simulink model "SNAP_DETUMBLE_HighPassFilter"  (R2024a)
settings: Solver=ode45  StartTime=0.0  StopTime=SNAP_sim_length  FixedStep=0.1  MaxStep=0.01  RelTol=1e-2  EnableMultiTasking=on
InitFcn:
  | SNAP_Simulink_Init_Function
values from neighbouring files (symbols this model uses):
  bias = [28.8675 28.8675 28.8675]    [SNAP_Simulink_Init_Function.m]    (also in Script_magnetorquer_and_magnetometer.m; SnapParameters.m)
  boira_Imax = boira_max_magnetic_torque./boira_magnetic_gains    [SNAP_Simulink_Init_Function.m]    (also in Script_magnetorquer_and_magnetometer.m; SnapParameters.m)
  boira_magnetic_gains = [2.3 2.3 2.1]    [SNAP_Simulink_Init_Function.m]    (also in Script_magnetorquer_and_magnetometer.m; SnapParameters.m)
  day = C - E + F - floor(30.6001 * G)    [julian2datetime.m]
  EN_2BodyModel = 1    [SNAP_Simulink_Init_Function.m]
  EN_Aero = SNAP_sim_params.aero_enabled    [SNAP_Simulink_Init_Function.m]
  EN_GG = 1    [SNAP_Simulink_Init_Function.m]
  EN_Hyst = 0    [SNAP_Simulink_Init_Function.m]
  EN_Mag = 1    [SNAP_Simulink_Init_Function.m]
  initial_position = SNAP_sim_params.initial_position    [SNAP_Simulink_Init_Function.m]
  initial_velocity = SNAP_sim_params.initial_velocity    [SNAP_Simulink_Init_Function.m]
  lookup_breakpoints_mmeter = linspace(-200,200,50)*10^3    [SNAP_Simulink_Init_Function.m]    (also in Script_magnetorquer_and_magnetometer.m; SnapParameters.m)
  lookup_breakpoints_mtorquer = linspace(-boira_Imax(1)*2,boira_Imax(1)*2,55)    [SNAP_Simulink_Init_Function.m]    (also in Script_magnetorquer_and_magnetometer.m; SnapParameters.m)
  lookup_tabledata_mmeter = lookup_breakpoints_mmeter+max_deviation_mmeter*sin(pi*lookup_breakpoints_mmeter/max_breakpoint_mmeter)    [SNAP_Simulink_Init_Function.m]    (also in Script_magnetorquer_and_magnetometer.m; SnapParameters.m)
  lookup_tabledata_mtorquer = lookup_breakpoints_mtorquer+max_deviation_mtorquer*sin(pi*lookup_breakpoints_mtorquer/max_breakpoint_mtorquer)    [SNAP_Simulink_Init_Function.m]    (also in Script_magnetorquer_and_magnetometer.m; SnapParameters.m)
  noise = 0    [SNAP_Simulink_Init_Function.m]    (also in Script_magnetorquer_and_magnetometer.m; SnapParameters.m)
  noise_variance = 30    [SNAP_Simulink_Init_Function.m]    (also in Script_magnetorquer_and_magnetometer.m; SnapParameters.m)
  rotm_mmeter = eul2rotm([missalingment_x_mmeter missalingment_y_mmeter missalingment_z_mmeter])    [SNAP_Simulink_Init_Function.m]    (also in Script_magnetorquer_and_magnetometer.m; SnapParameters.m)
  rotm_mtorquer = eul2rotm([missalingment_x_mtorquer missalingment_y_mtorquer missalingment_z_mtorquer])    [SNAP_Simulink_Init_Function.m]    (also in Script_magnetorquer_and_magnetometer.m; SnapParameters.m)
  second = (day_fraction - hour - minute / 60) * 3600    [julian2datetime.m]
  SNAP_Br = SNAP_sim_params.Br    [SNAP_Simulink_Init_Function.m]
  SNAP_Bs = SNAP_sim_params.Bs    [SNAP_Simulink_Init_Function.m]
  SNAP_CONST_a3H0 = 7.943e15    (= 7.943e+15)    [SNAP_Simulink_Init_Function.m]
  SNAP_CONST_earth_mag_dipole = [sin(168.6*pi/180)* cos(109.3*pi/180), sin(168.6*pi/180)* sin(109.3*pi/180), cos(168.6*pi/180)]    [SNAP_Simulink_Init_Function.m]
  SNAP_CONST_G_earth = 6.6742e-11    [SNAP_Simulink_Init_Function.m]
  SNAP_CONST_m_earth = 5.9736e24    (= 5.9736e+24)    [SNAP_Simulink_Init_Function.m]
  SNAP_CONST_mu0 = 4*pi*1e-7    (= 1.25663706144e-06)    [SNAP_Simulink_Init_Function.m]
  SNAP_CONST_r_earth = 6.36101e6    (= 6361010)    [SNAP_Simulink_Init_Function.m]
  SNAP_Hc = SNAP_sim_params.Hc    [SNAP_Simulink_Init_Function.m]
  SNAP_init_rates = SNAP_sim_params.init_rates    [SNAP_Simulink_Init_Function.m]
  SNAP_JD = SNAP_sim_params.JD    [SNAP_Simulink_Init_Function.m]
  SNAP_sat_inertia = boira_inertia    [SNAP_Simulink_Init_Function.m]
  SNAP_sat_mass = boira_mass    (= 2)    [SNAP_Simulink_Init_Function.m]
  SNAP_starting_ECI2ECEF_dcm = dcmeci2ecef('IAU-2000/2006',SNAP_sim_params.DateVector)    [SNAP_Simulink_Init_Function.m]
  SNAP_V_hyst = boira_V_hyst    [SNAP_Simulink_Init_Function.m]
undefined symbols (not defined in the file or in its folder): aeroCIP2006, magnitude, SNAPaero
libraries: vrlib x22, sharedtransform x9, simulink x9, aerolibutil x6, aerolibconvert2 x5, aerolibobsolete x1, aerolibanim x1, matrix_library x1
(part 2 of 2)

== system SNAP_DETUMBLE_HighPassFilter/Magnets/Eearth L-Shell Magnetic Model/ECEF2ECI ==
  ECEF : Inport
  Constant1 : Constant  Value=[0 0]
  Constant3 : Constant  Value=SNAP_starting_ECI2ECEF_dcm
  Gain1 : Gain  Gain=-1
  Math Function2 : Math  Operator=transpose  SignedPower=on
  Mux1 : Mux  Inputs=2
  Ramp2 : simulink/Sources/Ramp  slope="7.292115856e-5   %2*pi/(24*60*60)  %radians/second (one rotation per day )"  start=0  InitialOutput=0
  Rotation Angles to Direction Cosine Matrix1 : sharedtransform/Rotation Angles to Direction Cosine Matrix  rotationOrder=ZYX  aMode=aMode
  product 2 : Product  Multiplication=Matrix(*)  RndMeth=Zero
  product 4 : Product  Multiplication=Matrix(*)  RndMeth=Zero
  ECI : Outport
  wires:
  ECEF/1 -> product 4/1
  Ramp2/1 -> Gain1/1
  Gain1/1 -> Mux1/1
  Mux1/1 -> Rotation Angles to Direction Cosine Matrix1/1
  Constant1/1 -> Mux1/2
  product 2/1 -> Math Function2/1
  Rotation Angles to Direction Cosine Matrix1/1 -> product 2/2
  Constant3/1 -> product 2/1
  Math Function2/1 -> product 4/2
  product 4/1 -> ECI/1

== system SNAP_DETUMBLE_HighPassFilter/Magnets/Eearth L-Shell Magnetic Model/ECI2ECEF - position1 ==
  ECI : Inport
  Constant : Constant  Value=[0 0]
  Constant2 : Constant  Value=SNAP_starting_ECI2ECEF_dcm
  Gain : Gain  Gain=-1
  Mux : Mux  Inputs=2
  Ramp1 : simulink/Sources/Ramp  slope="7.292115856e-5   %2*pi/(24*60*60)  %radians/second (one rotation per day )"  start=0  InitialOutput=0
  Rotation Angles to Direction Cosine Matrix : sharedtransform/Rotation Angles to Direction Cosine Matrix  rotationOrder=ZYX  aMode=aMode
  product 1 : Product  Multiplication=Matrix(*)  RndMeth=Zero
  product 2 : Product  Multiplication=Matrix(*)  RndMeth=Zero
  ECEF : Outport
  wires:
  product 2/1 -> ECEF/1
  ECI/1 -> product 2/1
  Ramp1/1 -> Gain/1
  Gain/1 -> Mux/1
  Mux/1 -> Rotation Angles to Direction Cosine Matrix/1
  Constant/1 -> Mux/2
  product 1/1 -> product 2/2
  Rotation Angles to Direction Cosine Matrix/1 -> product 1/2
  Constant2/1 -> product 1/1

== system SNAP_DETUMBLE_HighPassFilter/ECI2ECEF - position/Direction Cosine Matrix ECI to ECEF1/IAUReduction/Additional Time Calculations ==
  ssUT : Inport
  "JD " : Inport  Port=2
  Bias : Bias  Bias=-51544.5  SaturateOnIntegerOverflow=off
  Constant : Constant
  Math Function : Math  Operator=mod  SignedPower=on
  Sum : Sum  Inputs=|++
  gainVal : Gain  Gain=1/86400
  jdElapsed : Outport
  jdFraction : Outport  Port=2
  wires:
  gainVal/1 -> Sum/2
  ssUT/1 -> gainVal/1
  "JD "/1 -> Sum/1
  Sum/1 -> Bias/1  "jdUT1"
  Bias/1 -> Math Function/1, jdElapsed/1
  Math Function/1 -> jdFraction/1
  Constant/1 -> Math Function/2

== system SNAP_DETUMBLE_HighPassFilter/ECI2ECEF - position/Direction Cosine Matrix ECI to ECEF1/IAUReduction/Celestial motion of the CIP ==
  "[dX,dY]" : Inport
  tTT : Inport  Port=2
  Lunisolar and planetary nutation : Subsystem
  P03 Precession : Subsystem
  Q : Outport
  wires:
  "[dX,dY]"/1 -> P03 Precession/1("[dX dY]")
  P03 Precession/1(Q) -> Q/1
  Lunisolar and planetary nutation/1(nutationV) -> P03 Precession/3(nutationV)
  tTT/1 -> P03 Precession/2(tTT), Lunisolar and planetary nutation/1(tTT)

== system SNAP_DETUMBLE_HighPassFilter/ECI2ECEF - position/Direction Cosine Matrix ECI to ECEF1/IAUReduction/Earth Rotation ==
  jdElapsed : Inport
  jdFraction : Inport  Port=2
  Bias1 : Bias  Bias=0.7790572732640  SaturateOnIntegerOverflow=off
  Constant : Constant  Value=2*pi
  Constant1 : Constant  Value=[0 0]
  Gain : Gain  Gain=0.00273781191135448
  Gain1 : Gain  Gain=2*pi
  Math Function : Math  Operator=mod  SignedPower=on
  Mux : Mux  Inputs=2
  Rotation Angles to Direction Cosine Matrix : sharedtransform/Rotation Angles to Direction Cosine Matrix  rotationOrder=ZYX  aMode=aMode
  Sum : Sum  Inputs=|++
  R : Outport
  wires:
  Mux/1 -> Rotation Angles to Direction Cosine Matrix/1
  Rotation Angles to Direction Cosine Matrix/1 -> R/1
  Constant1/1 -> Mux/2
  Math Function/1 -> Mux/1  "thetaERA"
  Gain1/1 -> Math Function/1
  jdElapsed/1 -> Gain/1
  jdFraction/1 -> Bias1/1
  Constant/1 -> Math Function/2
  Bias1/1 -> Sum/1
  Gain/1 -> Sum/2
  Sum/1 -> Gain1/1

== system SNAP_DETUMBLE_HighPassFilter/ECI2ECEF - position/Direction Cosine Matrix ECI to ECEF1/IAUReduction/Polar Motion ==
  tTT : Inport
  "[xp,yp]" : Inport  Port=2
  Angle Conversion : aerolibconvert2/Angle Conversion  IU=deg  OU=rad
  Demux : Demux  Outputs=2
  Gain : Gain  Gain=-0.000047/3600
  Gain1 : Gain  Gain=-1
  Mux : Mux  Inputs=3
  Rotation Angles to Direction Cosine Matrix : sharedtransform/Rotation Angles to Direction Cosine Matrix  rotationOrder=ZYX  aMode=aMode
  W : Outport
  wires:
  Rotation Angles to Direction Cosine Matrix/1 -> W/1
  Mux/1 -> Rotation Angles to Direction Cosine Matrix/1
  Gain/1 -> Angle Conversion/1
  tTT/1 -> Gain/1
  Angle Conversion/1 -> Mux/1  "sp"
  "[xp,yp]"/1 -> Gain1/1
  Gain1/1 -> Demux/1
  Demux/1 -> Mux/2
  Demux/2 -> Mux/3

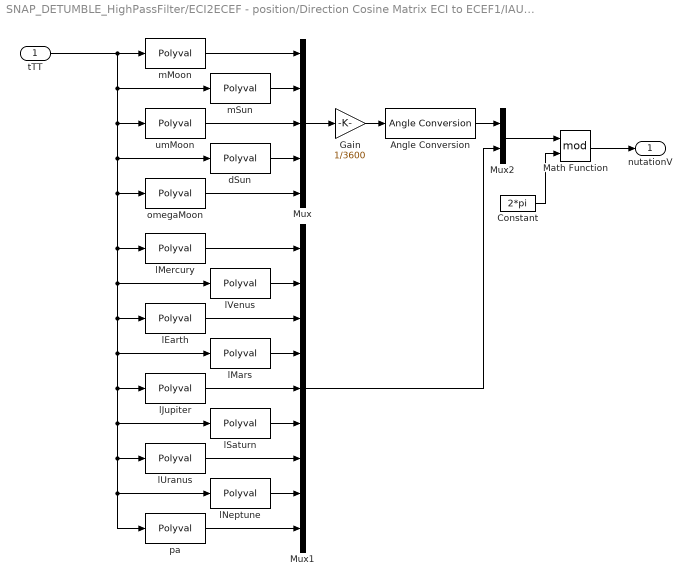
== system SNAP_DETUMBLE_HighPassFilter/ECI2ECEF - position/Direction Cosine Matrix ECI to ECEF1/IAUReduction/Celestial motion of the CIP/Lunisolar and planetary nutation ==
  tTT : Inport
  Angle Conversion : aerolibconvert2/Angle Conversion  IU=deg  OU=rad
  Constant : Constant  Value=2*pi
  Gain : Gain  Gain=1/3600
  Math Function : Math  Operator=mod  SignedPower=on
  Mux : Mux  Inputs=5
  Mux1 : Mux  Inputs=9
  Mux2 : Mux  Inputs=2
  dSun : Polyval  Coefs=[-0.00003169 0.006593 -6.3706 1602961601.2090 1072260.703692]
  lEarth : Polyval  Coefs=[628.3075849991 1.753470314]
  lJupiter : Polyval  Coefs=[52.9690962641 0.599546497]
  lMars : Polyval  Coefs=[334.06124267 6.203480913]
  lMercury : Polyval  Coefs=[2608.7903141574 4.402608842]
  lNeptune : Polyval  Coefs=[3.8133035638 5.311886287]
  lSaturn : Polyval  Coefs=[21.329910496 0.874016757]
  lUranus : Polyval  Coefs=[7.4781598567 5.481293872]
  lVenus : Polyval  Coefs=[1021.3285546211 3.176146697]
  mMoon : Polyval  Coefs=[-0.00024470 0.051635 31.8792 1717915923.2178 485868.249036]
  mSun : Polyval  Coefs=[-0.00001149 0.000136 -0.5532 129596581.0481 1287104.793048]
  omegaMoon : Polyval  Coefs=[-0.00005939 0.007702 7.4722 -6962890.5431 450160.398036]
  pa : Polyval  Coefs=[0.00000538691 0.02438175 0]
  umMoon : Polyval  Coefs=[0.00000417 -0.001037 -12.7512 1739527262.8478 335779.526232]
  nutationV : Outport
  wires:
  Mux1/1 -> Mux2/2
  pa/1 -> Mux1/9
  lNeptune/1 -> Mux1/8
  lUranus/1 -> Mux1/7
  lSaturn/1 -> Mux1/6
  lJupiter/1 -> Mux1/5
  lMars/1 -> Mux1/4
  Math Function/1 -> nutationV/1
  Constant/1 -> Math Function/2
  Mux2/1 -> Math Function/1
  Angle Conversion/1 -> Mux2/1
  lEarth/1 -> Mux1/3
  lVenus/1 -> Mux1/2
  lMercury/1 -> Mux1/1
  Gain/1 -> Angle Conversion/1
  Mux/1 -> Gain/1
  omegaMoon/1 -> Mux/5
  dSun/1 -> Mux/4
  umMoon/1 -> Mux/3
  mSun/1 -> Mux/2
  mMoon/1 -> Mux/1
  tTT/1 -> mMoon/1, mSun/1, umMoon/1, omegaMoon/1, lMercury/1, lEarth/1, lMars/1, lJupiter/1, lSaturn/1, lUranus/1, lNeptune/1, pa/1, lVenus/1, dSun/1

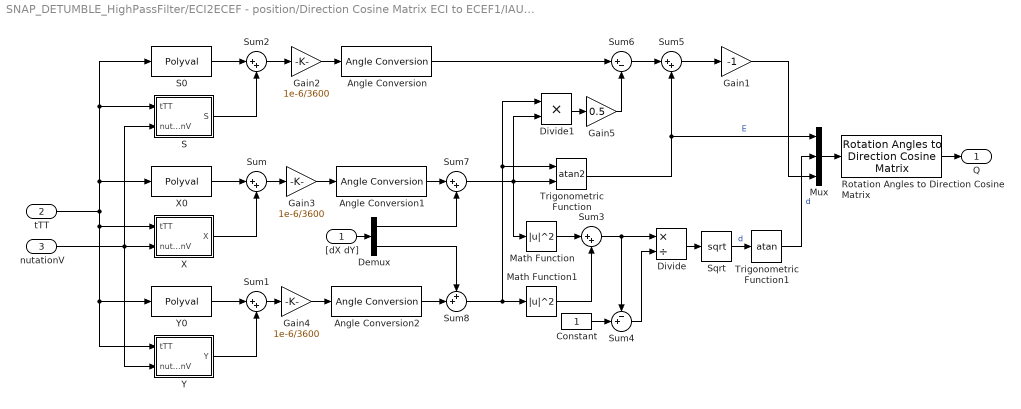
== system SNAP_DETUMBLE_HighPassFilter/ECI2ECEF - position/Direction Cosine Matrix ECI to ECEF1/IAUReduction/Celestial motion of the CIP/P03 Precession ==
  "[dX dY]" : Inport
  tTT : Inport  Port=2
  nutationV : Inport  Port=3
  Angle Conversion : aerolibconvert2/Angle Conversion  IU=deg  OU=rad
  Angle Conversion1 : aerolibconvert2/Angle Conversion  IU=deg  OU=rad
  Angle Conversion2 : aerolibconvert2/Angle Conversion  IU=deg  OU=rad
  Constant : Constant
  Demux : Demux  Outputs=2
  Divide : Product  Inputs=*/
  Divide1 : Product  Inputs=**
  Gain1 : Gain  Gain=-1
  Gain2 : Gain  Gain=1e-6/3600
  Gain3 : Gain  Gain=1e-6/3600
  Gain4 : Gain  Gain=1e-6/3600
  Gain5 : Gain  Gain=0.5
  Math Function : Math  Operator=magnitude^2  SignedPower=on
  Math Function1 : Math  Operator=magnitude^2  SignedPower=on
  Mux : Mux  Inputs=3
  Rotation Angles to Direction Cosine Matrix : sharedtransform/Rotation Angles to Direction Cosine Matrix  rotationOrder=ZYZ  aMode=aMode
  S : Subsystem
  S0 : Polyval  Coefs="[15.62 27.98 -72574.11 -122.68 3808.65  94]"
  Sqrt : Sqrt
  Sum{,1..3,5,7} (6 alike) : Sum  Inputs=|++
  Sum4 : Sum  Inputs=-+|
  Sum6 : Sum  Inputs=|+-
  Sum8 : Sum  Inputs=++|
  Trigonometric Function : Trigonometry  Operator=atan2
  Trigonometric Function1 : Trigonometry  Operator=atan
  X : Subsystem
  X0 : Polyval  Coefs=[5.9285 7.578 -198618.34 -429782.9 2004191898 -16617]
  Y : Subsystem
  Y0 : Polyval  Coefs=[0.1358 1112.526 1900.59 -22407274.7 -25896 -6951]
  Q : Outport
  wires:
  Trigonometric Function1/1 -> Mux/2  "d"
  Sqrt/1 -> Trigonometric Function1/1  "d"
  S/1(S) -> Sum2/2
  Y/1(Y) -> Sum1/2
  "[dX dY]"/1 -> Demux/1
  Sum6/1 -> Sum5/1
  Gain5/1 -> Sum6/2
  Divide1/1 -> Gain5/1
  Angle Conversion/1 -> Sum6/1
  Sum8/1 -> Math Function1/1, Trigonometric Function/1, Divide1/1
  Gain4/1 -> Angle Conversion2/1
  Gain3/1 -> Angle Conversion1/1
  Sum7/1 -> Trigonometric Function/2, Math Function/1, Divide1/2
  Gain2/1 -> Angle Conversion/1
  Rotation Angles to Direction Cosine Matrix/1 -> Q/1
  Mux/1 -> Rotation Angles to Direction Cosine Matrix/1
  Sum2/1 -> Gain2/1
  Trigonometric Function/1 -> Mux/1, Sum5/2  "E"
  Divide/1 -> Sqrt/1
  Sum4/1 -> Divide/2
  Constant/1 -> Sum4/2
  Sum3/1 -> Divide/1, Sum4/1
  Math Function1/1 -> Sum3/2
  Math Function/1 -> Sum3/1
  Sum/1 -> Gain3/1
  Sum1/1 -> Gain4/1
  S0/1 -> Sum2/1
  tTT/1 -> Y0/1, Y/1(tTT), X/1(tTT), S0/1, S/1(tTT), X0/1
  nutationV/1 -> S/2(nutationV), X/2(nutationV), Y/2(nutationV)
  Sum5/1 -> Gain1/1
  Gain1/1 -> Mux/3
  Y0/1 -> Sum1/1
  X/1(X) -> Sum/2
  X0/1 -> Sum/1
  Angle Conversion2/1 -> Sum8/2
  Demux/2 -> Sum8/1
  Angle Conversion1/1 -> Sum7/1
  Demux/1 -> Sum7/2

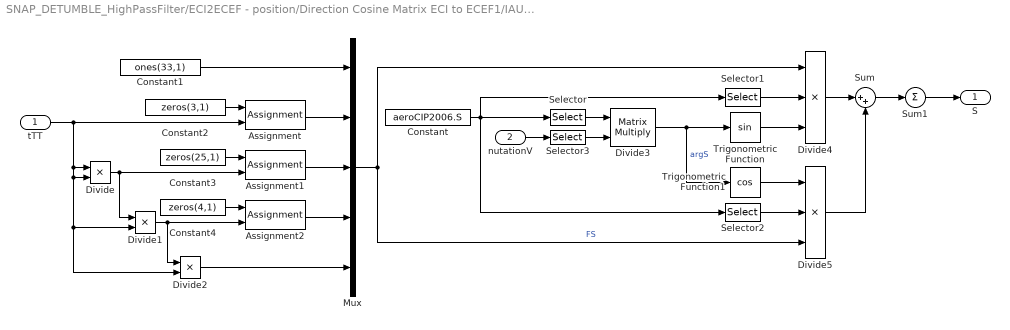
== system SNAP_DETUMBLE_HighPassFilter/ECI2ECEF - position/Direction Cosine Matrix ECI to ECEF1/IAUReduction/Celestial motion of the CIP/P03 Precession/S ==
  tTT : Inport
  nutationV : Inport  Port=2
  Assignment : Assignment  IndexOptions=Assign all  Indices=1  OutputSizes=1
  Assignment1 : Assignment  IndexOptions=Assign all  Indices=1  OutputSizes=1
  Assignment2 : Assignment  IndexOptions=Assign all  Indices=1  OutputSizes=1
  Constant : Constant  Value=aeroCIP2006.S
  Constant1 : Constant  Value=ones(33,1)
  Constant2 : Constant  Value=zeros(3,1)
  Constant3 : Constant  Value=zeros(25,1)
  Constant4 : Constant  Value=zeros(4,1)
  Divide : Product  Inputs=**
  Divide1 : Product  Inputs=**
  Divide2 : Product  Inputs=**
  Divide3 : Product  Inputs=**  Multiplication=Matrix(*)
  Divide4 : Product  Inputs=***
  Divide5 : Product  Inputs=***
  Mux : Mux  Inputs=5
  Selector : Selector  NumberOfDimensions=2  InputPortWidth=3  IndexOptions=Select all,Index vector (dialog)  Indices=[1 3],[4 5 6 7 8 9 10 11]  OutputSizes=1,11
  Selector1 : Selector  NumberOfDimensions=2  InputPortWidth=3  IndexOptions=Select all,Index vector (dialog)  Indices=[1 3],2  OutputSizes=1,14
  Selector2 : Selector  NumberOfDimensions=2  InputPortWidth=3  IndexOptions=Select all,Index vector (dialog)  Indices=[1 3],3  OutputSizes=1,14
  Selector3 : Selector  InputPortWidth=14  IndexOptions=Index vector (dialog)  Indices=[1 2 3 4 5 7 8 14]  OutputSizes=1
  Sum : Sum  Inputs=|++
  Sum1 : Sum  Inputs=|+|
  Trigonometric Function : Trigonometry
  Trigonometric Function1 : Trigonometry  Operator=cos
  S : Outport
  wires:
  Constant1/1 -> Mux/1
  Assignment/1 -> Mux/2
  Assignment1/1 -> Mux/3
  Assignment2/1 -> Mux/4
  Divide2/1 -> Mux/5
  Sum1/1 -> S/1
  Sum/1 -> Sum1/1
  Divide5/1 -> Sum/2
  Divide4/1 -> Sum/1
  Mux/1 -> Divide5/3, Divide4/1  "FS"
  Selector2/1 -> Divide5/2
  Trigonometric Function1/1 -> Divide5/1
  Selector1/1 -> Divide4/2
  Trigonometric Function/1 -> Divide4/3
  Divide3/1 -> Trigonometric Function/1, Trigonometric Function1/1  "argS"
  Constant/1 -> Selector2/1, Selector1/1, Selector/1
  Divide/1 -> Assignment1/2, Divide1/1
  Divide1/1 -> Assignment2/2, Divide2/1
  Constant4/1 -> Assignment2/1
  Constant3/1 -> Assignment1/1
  tTT/1 -> Assignment/2, Divide/1, Divide/2, Divide1/2, Divide2/2
  Constant2/1 -> Assignment/1
  nutationV/1 -> Selector3/1
  Selector3/1 -> Divide3/2
  Selector/1 -> Divide3/1

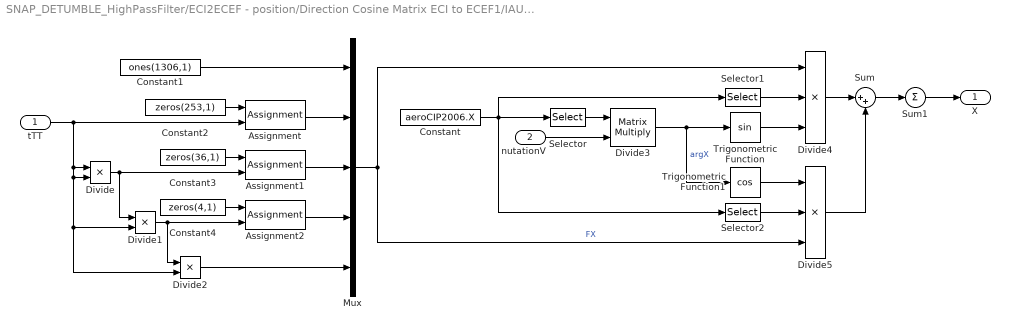
== system SNAP_DETUMBLE_HighPassFilter/ECI2ECEF - position/Direction Cosine Matrix ECI to ECEF1/IAUReduction/Celestial motion of the CIP/P03 Precession/X ==
  tTT : Inport
  nutationV : Inport  Port=2
  Assignment : Assignment  IndexOptions=Assign all  Indices=1  OutputSizes=1
  Assignment1 : Assignment  IndexOptions=Assign all  Indices=1  OutputSizes=1
  Assignment2 : Assignment  IndexOptions=Assign all  Indices=1  OutputSizes=1
  Constant : Constant  Value=aeroCIP2006.X
  Constant1 : Constant  Value=ones(1306,1)
  Constant2 : Constant  Value=zeros(253,1)
  Constant3 : Constant  Value=zeros(36,1)
  Constant4 : Constant  Value=zeros(4,1)
  Divide : Product  Inputs=**
  Divide1 : Product  Inputs=**
  Divide2 : Product  Inputs=**
  Divide3 : Product  Inputs=**  Multiplication=Matrix(*)
  Divide4 : Product  Inputs=***
  Divide5 : Product  Inputs=***
  Mux : Mux  Inputs=5
  Selector : Selector  NumberOfDimensions=2  InputPortWidth=3  IndexOptions=Select all,Starting index (dialog)  Indices=[1 3],4  OutputSizes=1,14
  Selector1 : Selector  NumberOfDimensions=2  InputPortWidth=3  IndexOptions=Select all,Index vector (dialog)  Indices=[1 3],2  OutputSizes=1,14
  Selector2 : Selector  NumberOfDimensions=2  InputPortWidth=3  IndexOptions=Select all,Index vector (dialog)  Indices=[1 3],3  OutputSizes=1,14
  Sum : Sum  Inputs=|++
  Sum1 : Sum  Inputs=|+|
  Trigonometric Function : Trigonometry
  Trigonometric Function1 : Trigonometry  Operator=cos
  X : Outport
  wires:
  Constant1/1 -> Mux/1
  Assignment/1 -> Mux/2
  Assignment1/1 -> Mux/3
  Assignment2/1 -> Mux/4
  Divide2/1 -> Mux/5
  Sum1/1 -> X/1
  Sum/1 -> Sum1/1
  Divide5/1 -> Sum/2
  Divide4/1 -> Sum/1
  Mux/1 -> Divide5/3, Divide4/1  "FX"
  Selector2/1 -> Divide5/2
  Trigonometric Function1/1 -> Divide5/1
  Selector1/1 -> Divide4/2
  Trigonometric Function/1 -> Divide4/3
  Divide3/1 -> Trigonometric Function/1, Trigonometric Function1/1  "argX"
  Selector/1 -> Divide3/1
  nutationV/1 -> Divide3/2
  Constant/1 -> Selector/1, Selector1/1, Selector2/1
  Divide/1 -> Assignment1/2, Divide1/1
  Divide1/1 -> Assignment2/2, Divide2/1
  Constant4/1 -> Assignment2/1
  Constant3/1 -> Assignment1/1
  tTT/1 -> Divide/1, Divide/2, Divide1/2, Divide2/2, Assignment/2
  Constant2/1 -> Assignment/1

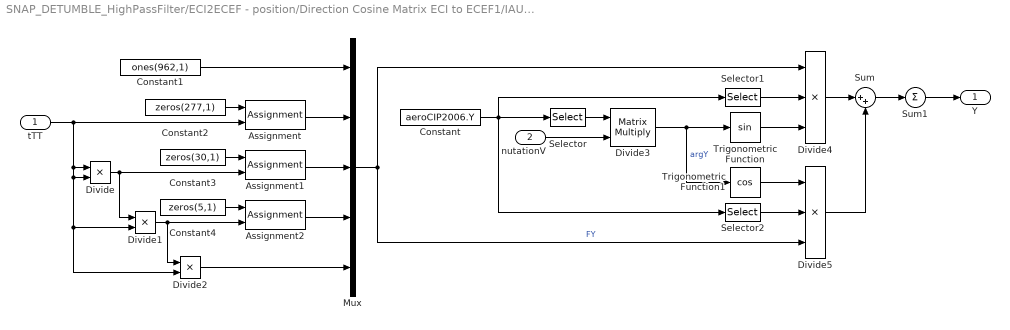
== system SNAP_DETUMBLE_HighPassFilter/ECI2ECEF - position/Direction Cosine Matrix ECI to ECEF1/IAUReduction/Celestial motion of the CIP/P03 Precession/Y ==
  tTT : Inport
  nutationV : Inport  Port=2
  Assignment : Assignment  IndexOptions=Assign all  Indices=1  OutputSizes=1
  Assignment1 : Assignment  IndexOptions=Assign all  Indices=1  OutputSizes=1
  Assignment2 : Assignment  IndexOptions=Assign all  Indices=1  OutputSizes=1
  Constant : Constant  Value=aeroCIP2006.Y
  Constant1 : Constant  Value=ones(962,1)
  Constant2 : Constant  Value=zeros(277,1)
  Constant3 : Constant  Value=zeros(30,1)
  Constant4 : Constant  Value=zeros(5,1)
  Divide : Product  Inputs=**
  Divide1 : Product  Inputs=**
  Divide2 : Product  Inputs=**
  Divide3 : Product  Inputs=**  Multiplication=Matrix(*)
  Divide4 : Product  Inputs=***
  Divide5 : Product  Inputs=***
  Mux : Mux  Inputs=5
  Selector : Selector  NumberOfDimensions=2  InputPortWidth=3  IndexOptions=Select all,Starting index (dialog)  Indices=[1 3],4  OutputSizes=1,14
  Selector1 : Selector  NumberOfDimensions=2  InputPortWidth=3  IndexOptions=Select all,Index vector (dialog)  Indices=[1 3],2  OutputSizes=1,14
  Selector2 : Selector  NumberOfDimensions=2  InputPortWidth=3  IndexOptions=Select all,Index vector (dialog)  Indices=[1 3],3  OutputSizes=1,14
  Sum : Sum  Inputs=|++
  Sum1 : Sum  Inputs=|+|
  Trigonometric Function : Trigonometry
  Trigonometric Function1 : Trigonometry  Operator=cos
  Y : Outport
  wires:
  Constant2/1 -> Assignment/1
  tTT/1 -> Assignment/2, Divide2/2, Divide1/2, Divide/2, Divide/1
  Constant3/1 -> Assignment1/1
  Constant4/1 -> Assignment2/1
  Divide1/1 -> Divide2/1, Assignment2/2
  Divide/1 -> Divide1/1, Assignment1/2
  Constant/1 -> Selector2/1, Selector1/1, Selector/1
  nutationV/1 -> Divide3/2
  Selector/1 -> Divide3/1
  Divide3/1 -> Trigonometric Function1/1, Trigonometric Function/1  "argY"
  Trigonometric Function/1 -> Divide4/3
  Selector1/1 -> Divide4/2
  Trigonometric Function1/1 -> Divide5/1
  Selector2/1 -> Divide5/2
  Mux/1 -> Divide4/1, Divide5/3  "FY"
  Divide4/1 -> Sum/1
  Divide5/1 -> Sum/2
  Sum/1 -> Sum1/1
  Sum1/1 -> Y/1
  Divide2/1 -> Mux/5
  Assignment2/1 -> Mux/4
  Assignment1/1 -> Mux/3
  Assignment/1 -> Mux/2
  Constant1/1 -> Mux/1

== matlab function SNAP_DETUMBLE_HighPassFilter/Hysteresis Material/Hysteresis Curve Model/Hysteresis Model ==
  data: B input; DBDT output; H input; DHDT input; Bsx input; Brx input; Hcx input
function DBDT = fcn(B, H, DHDT, Bsx, Brx, Hcx)
%#eml
mu0 = 4*pi*1e-7; 
% Bsx = 0.73 * 1e4;  %Tesla
% Brx = 0.35 * 1e4;
% Hcx = 1.59;  %A/m

k = 0.6;
p = 4.75;
q0 = 0.0885;

HL = tan(pi.*B./2./Bsx)./k - Hcx;

BP = 2 .* k .* Bsx/pi .* cos(pi*B/2/Bsx)*2;

F = (H-HL)/2/Hcx;

% neg = find(DHDT<0);
% F(neg) = 1-F(neg);

for i =1:3
    if(DHDT(i)<0)
        F(i) = 1-F(i);
    end
end


Q = q0 + (1-q0).*F.*p;

DBDT = Q.*BP.*DHDT;

% Based on this paper:
% "A MAGNETIC HYSTERESIS MODEL", Thomas W. Flatley, 1995
% http://ntrs.nasa.gov/archive/nasa/casi.ntrs.nasa.gov/19950021380_1995121380.pdf

== matlab function SNAP_DETUMBLE_HighPassFilter/MAGNETORQUER MODEL/MATLAB Function ==
  data: tau input; m output; B input
function m = required_magnetic_moment(tau,B)
% This function solves the equation system required to obtain the magnetic
% moment needed to produce a torque, tau in the presence of a magnetic
% field, B.

tau_closest = tau - B*(dot(tau, B)/dot(B, B));
W = B(1)*tau_closest(3)/B(2) + B(3)*tau_closest(2)/B(1) + B(3)*B(3)*tau_closest(3)/(B(2)*B(1));
Q = B(1)*B(1)/B(2) + B(2) + B(3)*B(3)/B(2);

m_2 = -W/Q;
m_1 = (tau_closest(3) + m_2*B(1))/B(2);
m_3 = (tau_closest(2) + m_1*B(3))/B(1);

m = [m_1;m_2;m_3];
end
